simulink model "Project_Open_Loop_v1"  (R2016a)
settings: Solver=VariableStepAuto  StartTime=0.0  StopTime=10.0  RelTol=1e-3
libraries: powerlib x10, powerlib_meascontrol x1
settings Model: Creator=Seo  LastModifiedBy=Seo

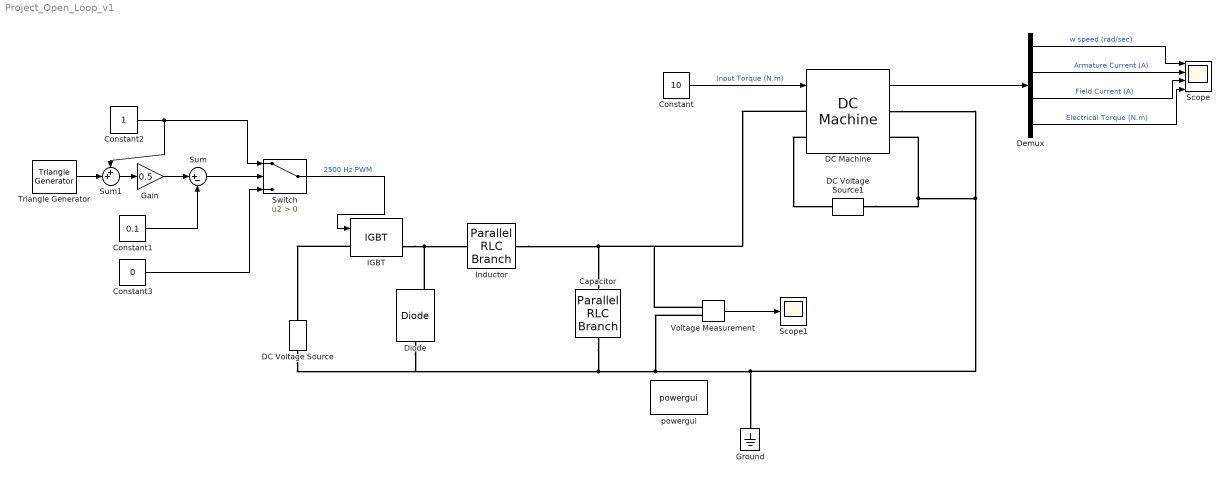
== system Project_Open_Loop_v1 ==
  Capacitor : powerlib/Elements/Parallel RLC Branch  LConnTagsString=a  RConnTagsString=__new0  BranchType=C  Resistance=1  Inductance=1e-3  SetiL0=off  InitialCurrent=0  Capacitance=1e-5  Setx0=off  InitialVoltage=0  Measurements=None
  Constant : Constant  Value=10
  Constant1 : Constant  Value=0.1
  Constant2 : Constant
  Constant3 : Constant  Value=0
  DC Machine : powerlib/Machines/DC Machine  PresetModel=No  MechanicalLoad=Torque TL  FieldType=Wound  ShowDetailedParameters=on  MeasurementBus=off  RLa="[ 0.6  0.012]"  RLf="[ 240  120]"  Laf=1.8  MachineConstant=Torque constant (N.m/A)  Ke=1.8  Kt=1.8  J=1  Bm=0  Tf=0  w0=1  Ifinit=1  TsPowergui=0  TsBlock=-1
  DC Voltage Source : powerlib/Electrical Sources/DC Voltage Source  Amplitude=300  Measurements=None
  DC Voltage Source1 : powerlib/Electrical Sources/DC Voltage Source  Amplitude=200  Measurements=None
  Demux : Demux
  Diode : powerlib/Power Electronics/Diode  Ron=0.001  Lon=0  Vf=0.8  IC=0  UseSnubber=off  Rs=500  Cs=250e-9  Measurements=on
  Gain : Gain  Gain=0.5
  Ground : powerlib/Elements/Ground  LConnTagsString=a
  IGBT : powerlib/Power Electronics/IGBT  Ron=0.001  Lon=0  Vf=1  Tf=1e-6  Tt=2e-6  IC=0  Rs=1e5  Cs=inf  Measurements=on
  Inductor : powerlib/Elements/Parallel RLC Branch  LConnTagsString=a  RConnTagsString=__new0  BranchType=L  Resistance=inf  Inductance=1e-3  SetiL0=off  InitialCurrent=0  Capacitance=0  Setx0=off  InitialVoltage=0  Measurements=None
  Scope : Scope  NumInputPorts=4
  Scope1 : Scope
  Sum : Sum  Inputs=|+-
  Sum1 : Sum  Inputs=++|
  Switch : Switch  Criteria=u2 > Threshold
  Triangle Generator : powerlib_meascontrol/Pulse & Signal Generators/Triangle Generator  Freq=2500  Phase=0  Ts=0
  Voltage Measurement : powerlib/Measurements/Voltage Measurement  PhasorSimulation=off  OutputType=Complex  PSBequivalent=0
  powergui : powerlib/powergui  Priority=1  SimulationMode=Continuous  SolverType=Tustin/Backward Euler (TBE)  SampleTime=50e-6  frequency=60  SPID=off  DisableSnubberDevices=off  DisableRonSwitches=off  DisableVfSwitches=off  SwTol=0  DisplayEquations=off  Interpol=off  ExternalGateDelay=off  methode=off  Ts=10  FunctionMessages=off  echomessages=off  HookPort=off  EnableUseOfTLC=off  x0status=blocks  frequencyindice=0  Pbase=100e6  ErrMax=1e-4  Iterations=50  UnitsV=kV  UnitsW=MW  buscounter=0  RestoreLinks=warning  ResistiveCurrentMeasurement=off  Frange=[0:2:500]  Ylog=off  Xlog=on  ShowGrid=off  save=off  variable=ZData  structure=0  ZoomFFT=off  StartTime=0.0  cycles=1  DisplayStyle=1  fundamental=60  FreqAxis=off  MaxFrequency=1000  frequencyindicesteady=1  RmsSteady=1  display=off
  wires:
  DC Machine/1 -> Demux/1
  Demux/1 -> Scope/1  "w speed (rad/sec)"
  Demux/2 -> Scope/2  "Armature Current (A)"
  Demux/3 -> Scope/3  "Field Current (A)"
  Demux/4 -> Scope/4  "Electrical Torque (N.m)"
  Constant/1 -> DC Machine/1  "Input Torque (N.m)"
  Sum/1 -> Switch/2
  Constant1/1 -> Sum/2
  Constant3/1 -> Switch/3
  Constant2/1 -> Sum1/1, Switch/1
  Switch/1 -> IGBT/1  "2500 Hz PWM"
  Sum1/1 -> Gain/1
  Triangle Generator/1 -> Sum1/2
  Gain/1 -> Sum/1
  Voltage Measurement/1 -> Scope1/1
  connections:
  DC Voltage Source1/LConn1 -- Voltage Measurement/LConn2 -- DC Voltage Source/LConn1 -- Diode/LConn1 -- Capacitor/RConn1 -- Ground/LConn1 -- DC Machine/RConn1 -- DC Machine/RConn2
  Inductor/RConn1 -- DC Machine/LConn1 -- Voltage Measurement/LConn1 -- Capacitor/LConn1
  Diode/RConn1 -- Inductor/LConn1 -- IGBT/RConn1
  IGBT/LConn1 -- DC Voltage Source/RConn1
  DC Machine/LConn2 -- DC Voltage Source1/RConn1
